simulink library "ATCC"  (R2025a)
settings: Solver=VariableStepAuto  StartTime=0.0  StopTime=10.0  RelTol=1e-3
undefined symbols (not defined in the file or in its folder): raptor_xcp_function, StateCAN
libraries: Utilities x44, Raptor_lib x16, simulink x2
settings Model: Creator=hyuga  LastModifiedBy=hyuga

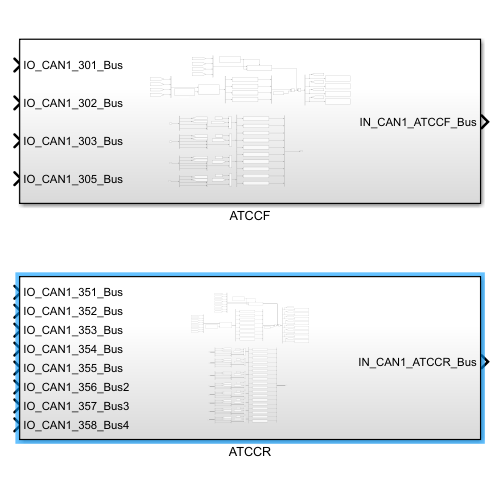
[thumbnail: Simulink's stored preview of the top-level diagram]
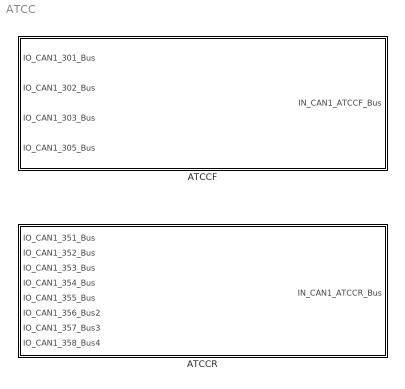
== system ATCC ==
  ATCCF : Subsystem
  ATCCR : Subsystem

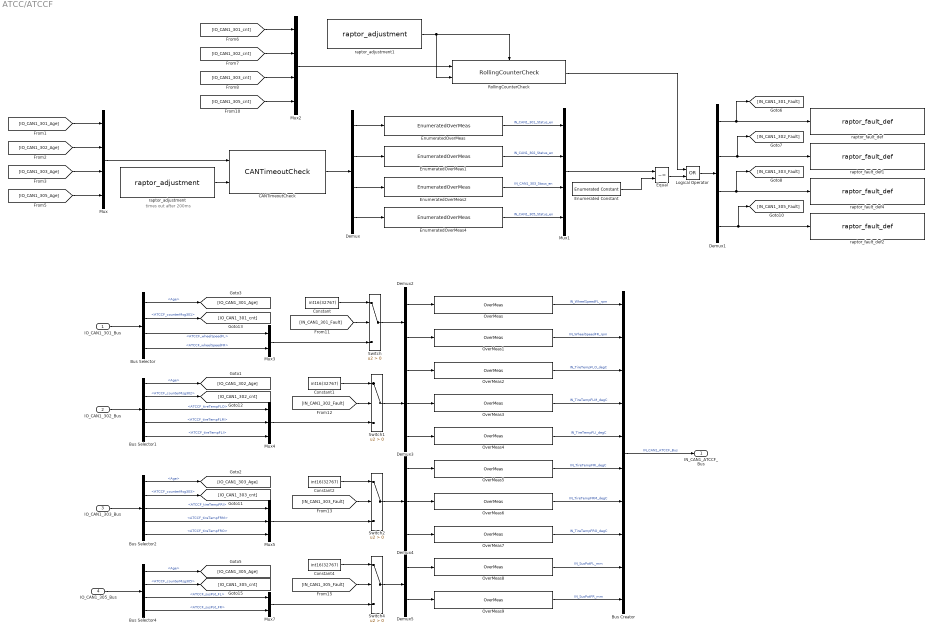
== system ATCC/ATCCF ==
  note: times out after 200ms
  IO_CAN1_301_Bus : Inport
  IO_CAN1_302_Bus : Inport  Port=2
  IO_CAN1_303_Bus : Inport  Port=3
  IO_CAN1_305_Bus : Inport  Port=4
  Bus Creator : BusCreator  Inputs=10
  Bus Selector : BusSelector  OutputSignals=Age,ATCCF_counterMsg301,ATCCF_wheelSpeedFL,ATCCF_wheelSpeedFR
  Bus Selector1 : BusSelector  OutputSignals=Age,ATCCF_counterMsg302,ATCCF_tireTempFLO,ATCCF_tireTempFLM,ATCCF_tireTempFLI
  Bus Selector2 : BusSelector  OutputSignals=Age,ATCCF_counterMsg303,ATCCF_tireTempFRI,ATCCF_tireTempFRM,ATCCF_tireTempFRO
  Bus Selector4 : BusSelector  OutputSignals=Age,ATCCF_counterMsg305,ATCCF_susPot_FL,ATCCF_susPot_FR
  CANTimeoutCheck : Utilities/CANTimeoutCheck
  Constant{,1..2,4} (4 alike) : Constant  Value=int16(32767)
  Demux : Demux
  Demux1 : Demux
  Demux2 : Demux  Outputs=2
  Demux3 : Demux  Outputs=3
  Demux4 : Demux  Outputs=3
  Demux5 : Demux  Outputs=2
  Enumerated Constant : simulink/Sources/Enumerated Constant  OutDataTypeStr=Enum: StateCAN  Value=StateCAN.Normal  SampleTime=inf
  EnumeratedOverMeas : Utilities/EnumeratedOverMeas  sigName='IN_CAN1_301_Status_en'  enumName='StateCAN'
  EnumeratedOverMeas1 : Utilities/EnumeratedOverMeas  sigName='IN_CAN1_302_Status_en'  enumName='StateCAN'
  EnumeratedOverMeas2 : Utilities/EnumeratedOverMeas  sigName='IN_CAN1_303_Staus_en'  enumName='StateCAN'
  EnumeratedOverMeas4 : Utilities/EnumeratedOverMeas  sigName='IN_CAN1_305_Status_en'  enumName='StateCAN'
  Equal : RelationalOperator  Operator=~=  OutDataTypeStr=boolean  RndMeth=Simplest  InputSameDT=off
  Logical Operator : Logic  Operator=OR  AllPortsSameDT=off  OutDataTypeStr=boolean
  Mux : Mux
  Mux1 : Mux
  Mux2 : Mux
  Mux3 : Mux  Inputs=2
  Mux4 : Mux  Inputs=3
  Mux5 : Mux  Inputs=3
  Mux7 : Mux  Inputs=2
  OverMeas : Utilities/OverMeas  sigName='IN_WheelSpeedFL_rpm'  minimum=-inf  maximum=inf
  OverMeas1 : Utilities/OverMeas  sigName='IN_WheelSpeedFR_rpm'  minimum=-inf  maximum=inf
  OverMeas2 : Utilities/OverMeas  sigName='IN_TireTempFLO_degC'  minimum=-inf  maximum=inf
  OverMeas3 : Utilities/OverMeas  sigName='IN_TireTempFLM_degC'  minimum=-inf  maximum=inf
  OverMeas4 : Utilities/OverMeas  sigName='IN_TireTempFLI_degC'  minimum=-inf  maximum=inf
  OverMeas5 : Utilities/OverMeas  sigName='IN_TireTempFRI_degC'  minimum=-inf  maximum=inf
  OverMeas6 : Utilities/OverMeas  sigName='IN_TireTempFRM_degC'  minimum=-inf  maximum=inf
  OverMeas7 : Utilities/OverMeas  sigName='IN_TireTempFRO_degC'  minimum=-inf  maximum=inf
  OverMeas8 : Utilities/OverMeas  sigName='IN_SusPotFL_mm'  minimum=-inf  maximum=inf
  OverMeas9 : Utilities/OverMeas  sigName='IN_SusPotFR_mm'  minimum=-inf  maximum=inf
  RollingCounterCheck : Utilities/RollingCounterCheck
  Switch{,1..2,4} (4 alike) : Switch  Criteria=u2 > Threshold  SaturateOnIntegerOverflow=off  InputSameDT=off
  raptor_adjustment : Raptor_lib/Data Storage/raptor_adjustment  paramName='IN_ATCCFTOThresh_na'  nameSource=Parameter  initValue=20  dataType=int32  storage=Calibration  calDispType=Number  calEnum={'False', 'True'}  calGain=1.0  calOffset=0.0  calMax=inf  calMin=-inf  calFormat='-1'  calUnit=''  calHelp=''  calAccess=1  calFunction=raptor_xcp_function(gcb)  calDispHeaders=off  calColHeaders={'Col1' 'Col2' 'Col3'}  calRowHeaders={'Row1' 'Row2' 'Row3'}
      settings: SourceProductName=Raptor
  raptor_adjustment1 : Raptor_lib/Data Storage/raptor_adjustment  paramName='IN_ATCCFRollingCounterEnable'  nameSource=Parameter  initValue=1  dataType=boolean  storage=Calibration  calDispType=Number  calEnum={'False', 'True'}  calGain=1.0  calOffset=0.0  calMax=inf  calMin=-inf  calFormat='-1'  calUnit=''  calHelp=''  calAccess=1  calFunction=raptor_xcp_function(gcb)  calDispHeaders=off  calColHeaders={'Col1' 'Col2' 'Col3'}  calRowHeaders={'Row1' 'Row2' 'Row3'}
      settings: SourceProductName=Raptor
  raptor_fault_def : Raptor_lib/Faults/raptor_fault_def  faultName='IN_CAN1_301_Fault'  persist=on  sticky=off  emisRelated=off  permanent=off  singleTrip=off  clearMethod=Standard  xLimit=25  yLimit=50  calEnable=on  addDisable=off  calAccess=1  calFunction='System | FaultManager'
      settings: SourceProductName=Raptor
  raptor_fault_def1 : Raptor_lib/Faults/raptor_fault_def  faultName='IN_CAN1_302_Fault'  persist=on  sticky=off  emisRelated=off  permanent=off  singleTrip=off  clearMethod=Standard  xLimit=25  yLimit=50  calEnable=on  addDisable=off  calAccess=1  calFunction='System | FaultManager'
      settings: SourceProductName=Raptor
  raptor_fault_def2 : Raptor_lib/Faults/raptor_fault_def  faultName='IN_CAN1_305_Fault'  persist=on  sticky=off  emisRelated=off  permanent=off  singleTrip=off  clearMethod=Standard  xLimit=25  yLimit=50  calEnable=on  addDisable=off  calAccess=1  calFunction='System | FaultManager'
      settings: SourceProductName=Raptor
  raptor_fault_def4 : Raptor_lib/Faults/raptor_fault_def  faultName='IN_CAN1_303_Fault'  persist=on  sticky=off  emisRelated=off  permanent=off  singleTrip=off  clearMethod=Standard  xLimit=25  yLimit=50  calEnable=on  addDisable=off  calAccess=1  calFunction='System | FaultManager'
      settings: SourceProductName=Raptor
  IN_CAN1_ATCCF_Bus : Outport
  wires:
  Bus Creator/1 -> IN_CAN1_ATCCF_Bus/1  "IN_CAN1_ATCCF_Bus"
  Switch4/1 -> Demux5/1
  Demux5/1 -> OverMeas8/1
  Demux5/2 -> OverMeas9/1
  OverMeas8/1 -> Bus Creator/9  "IN_SusPotFL_mm"
  OverMeas9/1 -> Bus Creator/10  "IN_SusPotFR_mm"
  Switch2/1 -> Demux4/1
  Demux4/1 -> OverMeas5/1
  Demux4/2 -> OverMeas6/1
  Demux4/3 -> OverMeas7/1
  OverMeas5/1 -> Bus Creator/6  "IN_TireTempFRI_degC"
  OverMeas6/1 -> Bus Creator/7  "IN_TireTempFRM_degC"
  OverMeas7/1 -> Bus Creator/8  "IN_TireTempFRO_degC"
  OverMeas4/1 -> Bus Creator/5  "IN_TireTempFLI_degC"
  OverMeas3/1 -> Bus Creator/4  "IN_TireTempFLM_degC"
  OverMeas2/1 -> Bus Creator/3  "IN_TireTempFLO_degC"
  Demux3/3 -> OverMeas4/1
  Demux3/2 -> OverMeas3/1
  Demux3/1 -> OverMeas2/1
  Switch1/1 -> Demux3/1
  OverMeas1/1 -> Bus Creator/2  "IN_WheelSpeedFR_rpm"
  OverMeas/1 -> Bus Creator/1  "IN_WheelSpeedFL_rpm"
  Demux2/2 -> OverMeas1/1
  Demux2/1 -> OverMeas/1
  Switch/1 -> Demux2/1
  Mux7/1 -> Switch4/3
  [IN_CAN1_305_Fault] -> Switch4/2
  Constant4/1 -> Switch4/1
  Bus Selector4/4 -> Mux7/2  "<ATCCF_susPot_FR>"
  Bus Selector4/3 -> Mux7/1  "<ATCCF_susPot_FL>"
  Mux5/1 -> Switch2/3
  [IN_CAN1_303_Fault] -> Switch2/2
  Constant2/1 -> Switch2/1
  Mux4/1 -> Switch1/3
  Constant1/1 -> Switch1/1
  [IN_CAN1_302_Fault] -> Switch1/2
  [IN_CAN1_301_Fault] -> Switch/2
  Constant/1 -> Switch/1
  Mux3/1 -> Switch/3
  raptor_adjustment1/1 -> RollingCounterCheck/2, RollingCounterCheck/Enable
  [IO_CAN1_301_cnt] -> Mux2/1
  [IO_CAN1_303_cnt] -> Mux2/3
  [IO_CAN1_305_cnt] -> Mux2/4
  Mux2/1 -> RollingCounterCheck/1
  [IO_CAN1_302_cnt] -> Mux2/2
  RollingCounterCheck/1 -> Logical Operator/1
  Equal/1 -> Logical Operator/2
  Logical Operator/1 -> Demux1/1
  Bus Selector4/2 -> [IO_CAN1_305_cnt]  "<ATCCF_counterMsg305>"
  Bus Selector1/5 -> Mux4/3  "<ATCCF_tireTempFLI>"
  Bus Selector1/4 -> Mux4/2  "<ATCCF_tireTempFLM>"
  Bus Selector1/3 -> Mux4/1  "<ATCCF_tireTempFLO>"
  Bus Selector2/5 -> Mux5/3  "<ATCCF_tireTempFRO>"
  Bus Selector2/4 -> Mux5/2  "<ATCCF_tireTempFRM>"
  Bus Selector2/3 -> Mux5/1  "<ATCCF_tireTempFRI>"
  Bus Selector2/2 -> [IO_CAN1_303_cnt]  "<ATCCF_counterMsg303>"
  Bus Selector1/2 -> [IO_CAN1_302_cnt]  "<ATCCF_counterMsg302>"
  Bus Selector/4 -> Mux3/2  "<ATCCF_wheelSpeedFR>"
  Bus Selector/3 -> Mux3/1  "<ATCCF_wheelSpeedFL>"
  Bus Selector/2 -> [IO_CAN1_301_cnt]  "<ATCCF_counterMsg301>"
  Demux1/2 -> raptor_fault_def1/1, [IN_CAN1_302_Fault]
  Demux1/4 -> raptor_fault_def2/1, [IN_CAN1_305_Fault]
  Demux1/3 -> raptor_fault_def4/1, [IN_CAN1_303_Fault]
  Demux1/1 -> raptor_fault_def/1, [IN_CAN1_301_Fault]
  Enumerated Constant/1 -> Equal/2
  Mux1/1 -> Equal/1
  EnumeratedOverMeas/1 -> Mux1/1  "IN_CAN1_301_Status_en"
  EnumeratedOverMeas1/1 -> Mux1/2  "IN_CAN1_302_Status_en"
  EnumeratedOverMeas2/1 -> Mux1/3  "IN_CAN1_303_Staus_en"
  EnumeratedOverMeas4/1 -> Mux1/4  "IN_CAN1_305_Status_en"
  Demux/4 -> EnumeratedOverMeas4/1
  Demux/3 -> EnumeratedOverMeas2/1
  Demux/2 -> EnumeratedOverMeas1/1
  Demux/1 -> EnumeratedOverMeas/1
  [IO_CAN1_302_Age] -> Mux/2
  CANTimeoutCheck/1 -> Demux/1
  raptor_adjustment/1 -> CANTimeoutCheck/2
  Mux/1 -> CANTimeoutCheck/1
  [IO_CAN1_305_Age] -> Mux/4
  [IO_CAN1_303_Age] -> Mux/3
  [IO_CAN1_301_Age] -> Mux/1
  Bus Selector4/1 -> [IO_CAN1_305_Age]  "<Age>"
  IO_CAN1_305_Bus/1 -> Bus Selector4/1
  Bus Selector2/1 -> [IO_CAN1_303_Age]  "<Age>"
  IO_CAN1_303_Bus/1 -> Bus Selector2/1
  Bus Selector1/1 -> [IO_CAN1_302_Age]  "<Age>"
  IO_CAN1_302_Bus/1 -> Bus Selector1/1
  Bus Selector/1 -> [IO_CAN1_301_Age]  "<Age>"
  IO_CAN1_301_Bus/1 -> Bus Selector/1

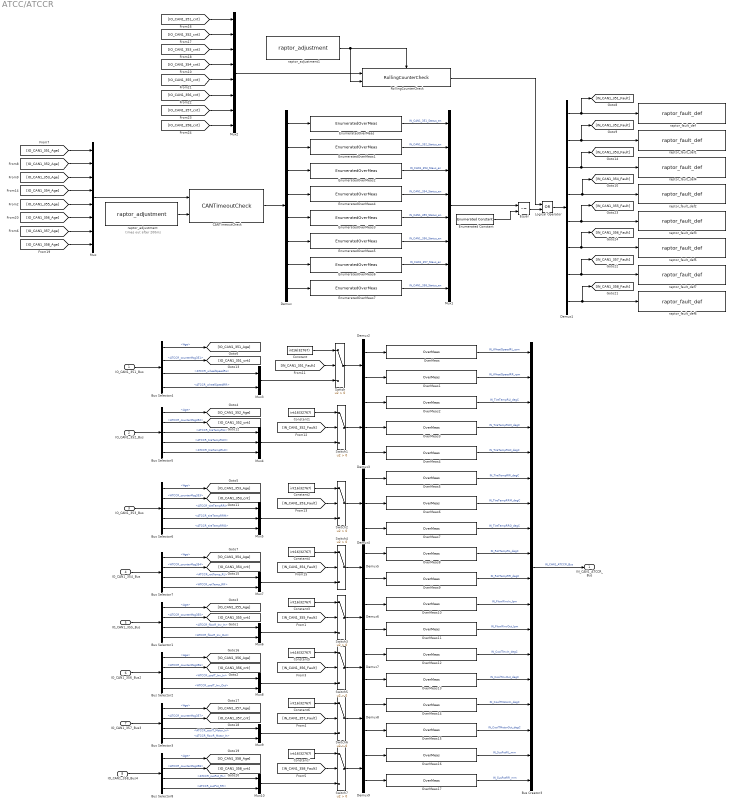
== system ATCC/ATCCR ==
  note: times out after 200ms
  IO_CAN1_351_Bus : Inport
  IO_CAN1_352_Bus : Inport  Port=2
  IO_CAN1_353_Bus : Inport  Port=3
  IO_CAN1_354_Bus : Inport  Port=4
  IO_CAN1_355_Bus : Inport  Port=5
  IO_CAN1_356_Bus2 : Inport  Port=6
  IO_CAN1_357_Bus3 : Inport  Port=7
  IO_CAN1_358_Bus4 : Inport  Port=8
  Bus Creator3 : BusCreator  Inputs=18
  Bus Selector1 : BusSelector  OutputSignals=Age,ATCCR_counterMsg355,ATCCR_flowR_Inv_In,ATCCR_flowR_Inv_Out
  Bus Selector2 : BusSelector  OutputSignals=Age,ATCCR_counterMsg356,ATCCR_coolT_Inv_In,ATCCR_coolT_Inv_Out
  Bus Selector3 : BusSelector  OutputSignals=Age,ATCCR_counterMsg357,ATCCR_coolT_Motor_In,ATCCR_flowR_Motor_In
  Bus Selector4 : BusSelector  OutputSignals=Age,ATCCR_counterMsg351,ATCCR_wheelSpeedRL,ATCCR_wheelSpeedRR
  Bus Selector5 : BusSelector  OutputSignals=Age,ATCCR_counterMsg352,ATCCR_tireTempRLI,ATCCR_tireTempRLM,ATCCR_tireTempRLO
  Bus Selector6 : BusSelector  OutputSignals=Age,ATCCR_counterMsg353,ATCCR_tireTempRRI,ATCCR_tireTempRRM,ATCCR_tireTempRRO
  Bus Selector7 : BusSelector  OutputSignals=Age,ATCCR_counterMsg354,ATCCR_rotTemp_RL,ATCCR_rotTemp_RR
  Bus Selector8 : BusSelector  OutputSignals=Age,ATCCR_counterMsg358,ATCCR_susPot_RL,ATCCR_susPot_RR
  CANTimeoutCheck : Utilities/CANTimeoutCheck
  Constant{,1..7} (8 alike) : Constant  Value=int16(32767)
  Demux : Demux  Outputs=8
  Demux1 : Demux  Outputs=8
  Demux{2,5..9} (6 alike) : Demux  Outputs=2
  Demux3 : Demux  Outputs=3
  Demux4 : Demux  Outputs=3
  Enumerated Constant : simulink/Sources/Enumerated Constant  OutDataTypeStr=Enum: StateCAN  Value=StateCAN.Normal  SampleTime=inf
  EnumeratedOverMeas : Utilities/EnumeratedOverMeas  sigName='IN_CAN1_351_Status_en'  enumName='StateCAN'
  EnumeratedOverMeas1 : Utilities/EnumeratedOverMeas  sigName='IN_CAN1_352_Status_en'  enumName='StateCAN'
  EnumeratedOverMeas2 : Utilities/EnumeratedOverMeas  sigName='IN_CAN1_353_Staus_en'  enumName='StateCAN'
  EnumeratedOverMeas3 : Utilities/EnumeratedOverMeas  sigName='IN_CAN1_355_Status_en'  enumName='StateCAN'
  EnumeratedOverMeas4 : Utilities/EnumeratedOverMeas  sigName='IN_CAN1_354_Status_en'  enumName='StateCAN'
  EnumeratedOverMeas5 : Utilities/EnumeratedOverMeas  sigName='IN_CAN1_356_Status_en'  enumName='StateCAN'
  EnumeratedOverMeas6 : Utilities/EnumeratedOverMeas  sigName='IN_CAN1_357_Staus_en'  enumName='StateCAN'
  EnumeratedOverMeas7 : Utilities/EnumeratedOverMeas  sigName='IN_CAN1_358_Status_en'  enumName='StateCAN'
  Equal : RelationalOperator  Operator=~=  OutDataTypeStr=boolean  RndMeth=Simplest  InputSameDT=off
  Logical Operator : Logic  Operator=OR  AllPortsSameDT=off  OutDataTypeStr=boolean
  Mux : Mux  Inputs=8
  Mux1 : Mux  Inputs=8
  Mux{3,6..10} (6 alike) : Mux  Inputs=2
  Mux2 : Mux  Inputs=8
  Mux4 : Mux  Inputs=3
  Mux5 : Mux  Inputs=3
  OverMeas : Utilities/OverMeas  sigName='IN_WheelSpeedRL_rpm'  minimum=-inf  maximum=inf
  OverMeas1 : Utilities/OverMeas  sigName='IN_WheelSpeedRR_rpm'  minimum=-inf  maximum=inf
  OverMeas10 : Utilities/OverMeas  sigName='IN_FlowRInvIn_lpm'  minimum=-inf  maximum=inf
  OverMeas11 : Utilities/OverMeas  sigName='IN_FlowRInvOut_lpm'  minimum=-inf  maximum=inf
  OverMeas12 : Utilities/OverMeas  sigName='IN_CoolTInvIn_degC'  minimum=-inf  maximum=inf
  OverMeas13 : Utilities/OverMeas  sigName='IN_CoolTInvOut_degC'  minimum=-inf  maximum=inf
  OverMeas14 : Utilities/OverMeas  sigName='IN_CoolTMotorIn_degC'  minimum=-inf  maximum=inf
  OverMeas15 : Utilities/OverMeas  sigName='IN_CoolTMotorOut_degC'  minimum=-inf  maximum=inf
  OverMeas16 : Utilities/OverMeas  sigName='IN_SusPotRL_mm'  minimum=-inf  maximum=inf
  OverMeas17 : Utilities/OverMeas  sigName='IN_SusPotRR_mm'  minimum=-inf  maximum=inf
  OverMeas2 : Utilities/OverMeas  sigName='IN_TireTempRLI_degC'  minimum=-inf  maximum=inf
  OverMeas3 : Utilities/OverMeas  sigName='IN_TireTempRLM_degC'  minimum=-inf  maximum=inf
  OverMeas4 : Utilities/OverMeas  sigName='IN_TireTempRLO_degC'  minimum=-inf  maximum=inf
  OverMeas5 : Utilities/OverMeas  sigName='IN_TireTempRRI_degC'  minimum=-inf  maximum=inf
  OverMeas6 : Utilities/OverMeas  sigName='IN_TireTempRRM_degC'  minimum=-inf  maximum=inf
  OverMeas7 : Utilities/OverMeas  sigName='IN_TireTempRRO_degC'  minimum=-inf  maximum=inf
  OverMeas8 : Utilities/OverMeas  sigName='IN_RotTempRL_degC'  minimum=-inf  maximum=inf
  OverMeas9 : Utilities/OverMeas  sigName='IN_RotTempRR_degC'  minimum=-inf  maximum=inf
  RollingCounterCheck : Utilities/RollingCounterCheck
  Switch{,1..7} (8 alike) : Switch  Criteria=u2 > Threshold  SaturateOnIntegerOverflow=off  InputSameDT=off
  raptor_adjustment : Raptor_lib/Data Storage/raptor_adjustment  paramName='IN_ATCCRTOThresh_na'  nameSource=Parameter  initValue=20  dataType=int32  storage=Calibration  calDispType=Number  calEnum={'False', 'True'}  calGain=1.0  calOffset=0.0  calMax=inf  calMin=-inf  calFormat='-1'  calUnit=''  calHelp=''  calAccess=1  calFunction=raptor_xcp_function(gcb)  calDispHeaders=off  calColHeaders={'Col1' 'Col2' 'Col3'}  calRowHeaders={'Row1' 'Row2' 'Row3'}
      settings: SourceProductName=Raptor
  raptor_adjustment1 : Raptor_lib/Data Storage/raptor_adjustment  paramName='IN_ATCCRRollingCounterEnable'  nameSource=Parameter  initValue=1  dataType=boolean  storage=Calibration  calDispType=Number  calEnum={'False', 'True'}  calGain=1.0  calOffset=0.0  calMax=inf  calMin=-inf  calFormat='-1'  calUnit=''  calHelp=''  calAccess=1  calFunction=raptor_xcp_function(gcb)  calDispHeaders=off  calColHeaders={'Col1' 'Col2' 'Col3'}  calRowHeaders={'Row1' 'Row2' 'Row3'}
      settings: SourceProductName=Raptor
  raptor_fault_def : Raptor_lib/Faults/raptor_fault_def  faultName='IN_CAN1_351_Fault'  persist=on  sticky=off  emisRelated=off  permanent=off  singleTrip=off  clearMethod=Standard  xLimit=25  yLimit=50  calEnable=on  addDisable=off  calAccess=1  calFunction='System | FaultManager'
      settings: SourceProductName=Raptor
  raptor_fault_def1 : Raptor_lib/Faults/raptor_fault_def  faultName='IN_CAN1_352_Fault'  persist=on  sticky=off  emisRelated=off  permanent=off  singleTrip=off  clearMethod=Standard  xLimit=25  yLimit=50  calEnable=on  addDisable=off  calAccess=1  calFunction='System | FaultManager'
      settings: SourceProductName=Raptor
  raptor_fault_def2 : Raptor_lib/Faults/raptor_fault_def  faultName='IN_CAN1_354_Fault'  persist=on  sticky=off  emisRelated=off  permanent=off  singleTrip=off  clearMethod=Standard  xLimit=25  yLimit=50  calEnable=on  addDisable=off  calAccess=1  calFunction='System | FaultManager'
      settings: SourceProductName=Raptor
  raptor_fault_def3 : Raptor_lib/Faults/raptor_fault_def  faultName='IN_CAN1_355_Fault'  persist=on  sticky=off  emisRelated=off  permanent=off  singleTrip=off  clearMethod=Standard  xLimit=25  yLimit=50  calEnable=on  addDisable=off  calAccess=1  calFunction='System | FaultManager'
      settings: SourceProductName=Raptor
  raptor_fault_def4 : Raptor_lib/Faults/raptor_fault_def  faultName='IN_CAN1_353_Fault'  persist=on  sticky=off  emisRelated=off  permanent=off  singleTrip=off  clearMethod=Standard  xLimit=25  yLimit=50  calEnable=on  addDisable=off  calAccess=1  calFunction='System | FaultManager'
      settings: SourceProductName=Raptor
  raptor_fault_def5 : Raptor_lib/Faults/raptor_fault_def  faultName='IN_CAN1_356_Fault'  persist=on  sticky=off  emisRelated=off  permanent=off  singleTrip=off  clearMethod=Standard  xLimit=25  yLimit=50  calEnable=on  addDisable=off  calAccess=1  calFunction='System | FaultManager'
      settings: SourceProductName=Raptor
  raptor_fault_def6 : Raptor_lib/Faults/raptor_fault_def  faultName='IN_CAN1_358_Fault'  persist=on  sticky=off  emisRelated=off  permanent=off  singleTrip=off  clearMethod=Standard  xLimit=25  yLimit=50  calEnable=on  addDisable=off  calAccess=1  calFunction='System | FaultManager'
      settings: SourceProductName=Raptor
  raptor_fault_def7 : Raptor_lib/Faults/raptor_fault_def  faultName='IN_CAN1_357_Fault'  persist=on  sticky=off  emisRelated=off  permanent=off  singleTrip=off  clearMethod=Standard  xLimit=25  yLimit=50  calEnable=on  addDisable=off  calAccess=1  calFunction='System | FaultManager'
      settings: SourceProductName=Raptor
  IN_CAN1_ATCCR_Bus : Outport
  wires:
  Bus Selector7/4 -> Mux7/2  "<ATCCR_rotTemp_RR>"
  Bus Selector7/3 -> Mux7/1  "<ATCCR_rotTemp_RL>"
  Bus Selector7/2 -> [IO_CAN1_354_cnt]  "<ATCCR_counterMsg354>"
  Bus Selector7/1 -> [IO_CAN1_354_Age]  "<Age>"
  Demux/8 -> EnumeratedOverMeas7/1
  Demux/7 -> EnumeratedOverMeas6/1
  Demux/6 -> EnumeratedOverMeas5/1
  Demux/5 -> EnumeratedOverMeas3/1
  EnumeratedOverMeas5/1 -> Mux1/6  "IN_CAN1_356_Status_en"
  EnumeratedOverMeas7/1 -> Mux1/8  "IN_CAN1_358_Status_en"
  EnumeratedOverMeas3/1 -> Mux1/5  "IN_CAN1_355_Status_en"
  EnumeratedOverMeas6/1 -> Mux1/7  "IN_CAN1_357_Staus_en"
  [IO_CAN1_358_cnt] -> Mux2/8
  [IO_CAN1_357_cnt] -> Mux2/7
  [IO_CAN1_356_cnt] -> Mux2/6
  [IO_CAN1_355_cnt] -> Mux2/5
  [IO_CAN1_356_Age] -> Mux/6
  [IO_CAN1_357_Age] -> Mux/7
  [IO_CAN1_358_Age] -> Mux/8
  Demux1/5 -> raptor_fault_def3/1, [IN_CAN1_355_Fault]
  Demux1/7 -> raptor_fault_def7/1, [IN_CAN1_357_Fault]
  Demux1/6 -> raptor_fault_def5/1, [IN_CAN1_356_Fault]
  Demux1/8 -> raptor_fault_def6/1, [IN_CAN1_358_Fault]
  Bus Selector8/4 -> Mux10/2  "<ATCCR_susPot_RR>"
  Bus Selector8/3 -> Mux10/1  "<ATCCR_susPot_RL>"
  Bus Selector8/2 -> [IO_CAN1_358_cnt]  "<ATCCR_counterMsg358>"
  [IN_CAN1_358_Fault] -> Switch7/2
  Mux10/1 -> Switch7/3
  Demux9/1 -> OverMeas16/1
  Switch7/1 -> Demux9/1
  OverMeas17/1 -> Bus Creator3/18  "IN_SusPotRR_mm"
  Bus Selector8/1 -> [IO_CAN1_358_Age]  "<Age>"
  Constant7/1 -> Switch7/1
  Demux9/2 -> OverMeas17/1
  OverMeas16/1 -> Bus Creator3/17  "IN_SusPotRL_mm"
  IO_CAN1_358_Bus4/1 -> Bus Selector8/1
  Bus Selector3/4 -> Mux9/2  "<ATCCR_flowR_Motor_In>"
  Bus Selector3/3 -> Mux9/1  "<ATCCR_coolT_Motor_In>"
  Bus Selector3/2 -> [IO_CAN1_357_cnt]  "<ATCCR_counterMsg357>"
  OverMeas14/1 -> Bus Creator3/15  "IN_CoolTMotorIn_degC"
  IO_CAN1_357_Bus3/1 -> Bus Selector3/1
  Demux8/2 -> OverMeas15/1
  Constant6/1 -> Switch6/1
  Bus Selector3/1 -> [IO_CAN1_357_Age]  "<Age>"
  OverMeas15/1 -> Bus Creator3/16  "IN_CoolTMotorOut_degC"
  Switch6/1 -> Demux8/1
  Demux8/1 -> OverMeas14/1
  Mux9/1 -> Switch6/3
  [IN_CAN1_357_Fault] -> Switch6/2
  Bus Selector2/4 -> Mux8/2  "<ATCCR_coolT_Inv_Out>"
  Bus Selector2/3 -> Mux8/1  "<ATCCR_coolT_Inv_In>"
  Bus Selector2/2 -> [IO_CAN1_356_cnt]  "<ATCCR_counterMsg356>"
  OverMeas13/1 -> Bus Creator3/14  "IN_CoolTInvOut_degC"
  Switch5/1 -> Demux7/1
  Mux8/1 -> Switch5/3
  [IN_CAN1_356_Fault] -> Switch5/2
  Demux7/1 -> OverMeas12/1
  OverMeas12/1 -> Bus Creator3/13  "IN_CoolTInvIn_degC"
  Constant5/1 -> Switch5/1
  Demux7/2 -> OverMeas13/1
  Bus Selector2/1 -> [IO_CAN1_356_Age]  "<Age>"
  IO_CAN1_356_Bus2/1 -> Bus Selector2/1
  [IO_CAN1_355_Age] -> Mux/5
  Demux6/2 -> OverMeas11/1
  Constant3/1 -> Switch3/1
  OverMeas10/1 -> Bus Creator3/11  "IN_FlowRInvIn_lpm"
  Bus Selector1/3 -> Mux6/1  "<ATCCR_flowR_Inv_In>"
  Demux6/1 -> OverMeas10/1
  Switch3/1 -> Demux6/1
  [IN_CAN1_355_Fault] -> Switch3/2
  OverMeas11/1 -> Bus Creator3/12  "IN_FlowRInvOut_lpm"
  Mux6/1 -> Switch3/3
  Bus Selector1/4 -> Mux6/2  "<ATCCR_flowR_Inv_Out>"
  Bus Selector1/1 -> [IO_CAN1_355_Age]  "<Age>"
  Bus Selector1/2 -> [IO_CAN1_355_cnt]  "<ATCCR_counterMsg355>"
  IO_CAN1_355_Bus/1 -> Bus Selector1/1
  Bus Selector6/5 -> Mux5/3  "<ATCCR_tireTempRRO>"
  Bus Selector6/4 -> Mux5/2  "<ATCCR_tireTempRRM>"
  Bus Selector6/3 -> Mux5/1  "<ATCCR_tireTempRRI>"
  Bus Selector6/2 -> [IO_CAN1_353_cnt]  "<ATCCR_counterMsg353>"
  Bus Selector5/5 -> Mux4/3  "<ATCCR_tireTempRLO>"
  Bus Selector5/4 -> Mux4/2  "<ATCCR_tireTempRLM>"
  Bus Selector5/3 -> Mux4/1  "<ATCCR_tireTempRLI>"
  Bus Selector5/2 -> [IO_CAN1_352_cnt]  "<ATCCR_counterMsg352>"
  Bus Selector4/4 -> Mux3/2  "<ATCCR_wheelSpeedRR>"
  Bus Selector4/3 -> Mux3/1  "<ATCCR_wheelSpeedRL>"
  Bus Selector4/2 -> [IO_CAN1_351_cnt]  "<ATCCR_counterMsg351>"
  [IN_CAN1_351_Fault] -> Switch/2
  Demux4/1 -> OverMeas5/1
  [IO_CAN1_352_Age] -> Mux/2
  Enumerated Constant/1 -> Equal/2
  OverMeas8/1 -> Bus Creator3/9  "IN_RotTempRL_degC"
  Constant4/1 -> Switch4/1
  [IO_CAN1_354_Age] -> Mux/4
  Demux2/1 -> OverMeas/1
  Demux2/2 -> OverMeas1/1
  Constant1/1 -> Switch1/1
  Demux3/1 -> OverMeas2/1
  Demux1/4 -> [IN_CAN1_354_Fault], raptor_fault_def2/1
  Demux4/3 -> OverMeas7/1
  Demux3/3 -> OverMeas4/1
  Demux/1 -> EnumeratedOverMeas/1
  [IN_CAN1_354_Fault] -> Switch4/2
  Bus Creator3/1 -> IN_CAN1_ATCCR_Bus/1  "IN_CAN1_ATCCR_Bus"
  Switch4/1 -> Demux5/1
  Mux7/1 -> Switch4/3
  Equal/1 -> Logical Operator/2
  IO_CAN1_352_Bus/1 -> Bus Selector5/1
  Mux4/1 -> Switch1/3
  OverMeas3/1 -> Bus Creator3/4  "IN_TireTempRLM_degC"
  Demux/2 -> EnumeratedOverMeas1/1
  [IO_CAN1_353_cnt] -> Mux2/3
  Switch1/1 -> Demux3/1
  Constant2/1 -> Switch2/1
  IO_CAN1_354_Bus/1 -> Bus Selector7/1
  Demux/3 -> EnumeratedOverMeas2/1
  RollingCounterCheck/1 -> Logical Operator/1
  [IO_CAN1_351_cnt] -> Mux2/1
  Bus Selector6/1 -> [IO_CAN1_353_Age]  "<Age>"
  OverMeas6/1 -> Bus Creator3/7  "IN_TireTempRRM_degC"
  CANTimeoutCheck/1 -> Demux/1
  Demux/4 -> EnumeratedOverMeas4/1
  [IO_CAN1_353_Age] -> Mux/3
  OverMeas5/1 -> Bus Creator3/6  "IN_TireTempRRI_degC"
  [IO_CAN1_354_cnt] -> Mux2/4
  OverMeas9/1 -> Bus Creator3/10  "IN_RotTempRR_degC"
  Mux3/1 -> Switch/3
  Demux1/2 -> raptor_fault_def1/1, [IN_CAN1_352_Fault]
  Demux1/3 -> [IN_CAN1_353_Fault], raptor_fault_def4/1
  [IO_CAN1_352_cnt] -> Mux2/2
  Bus Selector4/1 -> [IO_CAN1_351_Age]  "<Age>"
  OverMeas1/1 -> Bus Creator3/2  "IN_WheelSpeedRR_rpm"
  EnumeratedOverMeas2/1 -> Mux1/3  "IN_CAN1_353_Staus_en"
  IO_CAN1_353_Bus/1 -> Bus Selector6/1
  EnumeratedOverMeas/1 -> Mux1/1  "IN_CAN1_351_Status_en"
  Demux5/2 -> OverMeas9/1
  [IN_CAN1_352_Fault] -> Switch1/2
  OverMeas7/1 -> Bus Creator3/8  "IN_TireTempRRO_degC"
  raptor_adjustment1/1 -> RollingCounterCheck/Enable, RollingCounterCheck/2
  Demux5/1 -> OverMeas8/1
  Switch/1 -> Demux2/1
  OverMeas2/1 -> Bus Creator3/3  "IN_TireTempRLI_degC"
  Logical Operator/1 -> Demux1/1
  Mux1/1 -> Equal/1
  IO_CAN1_351_Bus/1 -> Bus Selector4/1
  OverMeas/1 -> Bus Creator3/1  "IN_WheelSpeedRL_rpm"
  raptor_adjustment/1 -> CANTimeoutCheck/2
  Bus Selector5/1 -> [IO_CAN1_352_Age]  "<Age>"
  Mux2/1 -> RollingCounterCheck/1
  Demux4/2 -> OverMeas6/1
  [IO_CAN1_351_Age] -> Mux/1
  OverMeas4/1 -> Bus Creator3/5  "IN_TireTempRLO_degC"
  Switch2/1 -> Demux4/1
  Constant/1 -> Switch/1
  EnumeratedOverMeas4/1 -> Mux1/4  "IN_CAN1_354_Status_en"
  Mux/1 -> CANTimeoutCheck/1
  Mux5/1 -> Switch2/3
  Demux3/2 -> OverMeas3/1
  Demux1/1 -> raptor_fault_def/1, [IN_CAN1_351_Fault]
  EnumeratedOverMeas1/1 -> Mux1/2  "IN_CAN1_352_Status_en"
  [IN_CAN1_353_Fault] -> Switch2/2
